simulink model "Three_Phase_180"  (R2019b)
settings: Solver=VariableStepAuto  StartTime=0.0  StopTime=0.1  RelTol=1e-3
libraries: powerlib x17
settings Model: Creator=swaga  LastModifiedBy=swaga
settings DataIOCC: ReturnWorkspaceOutputs=off

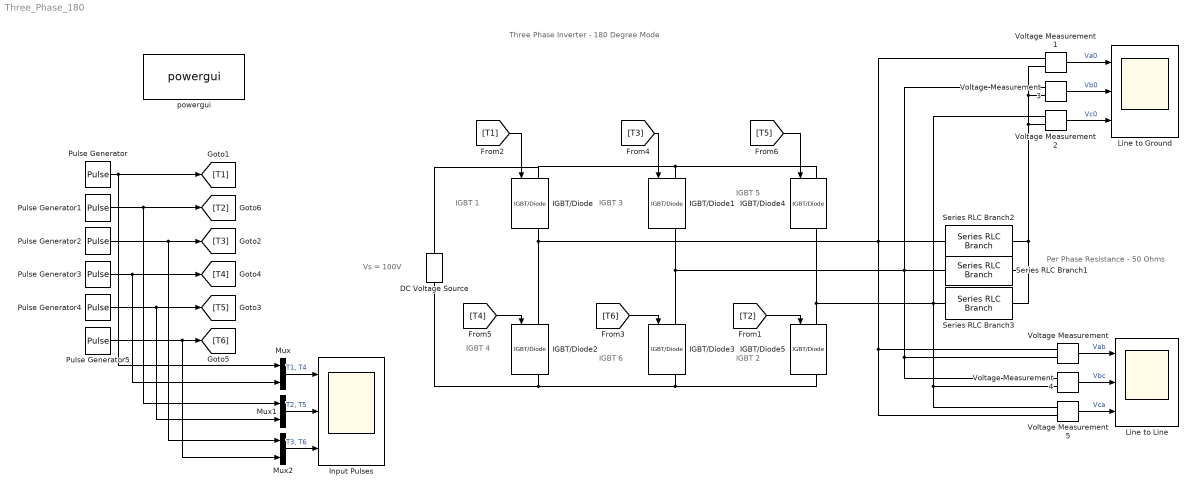
== system Three_Phase_180 ==
  note: Per Phase Resistance - 50 Ohms
  note: Vs = 100V
  note: IGBT 1
  note: Three Phase Inverter - 180 Degree Mode
  note: IGBT 3
  note: IGBT 4
  note: IGBT 6
  note: IGBT 5
  note: IGBT 2
  DC Voltage Source : powerlib/Electrical Sources/DC Voltage Source  Amplitude=100  Measurements=None
      settings: SourceProductName=Simscape Electrical
  IGBT/Diode{,1..5} (6 alike) : powerlib/Power Electronics/IGBT//Diode  Ron=1e-3  Rs=1e5  Cs=inf  Measurements=on
      settings: SourceProductName=Simscape Electrical
  Input Pulses : Scope  NumInputPorts=3
  "Line to Ground " : Scope  NumInputPorts=3
  Line to Line : Scope  NumInputPorts=3
  Mux : Mux  Inputs=2
  Mux1 : Mux  Inputs=2
  Mux2 : Mux  Inputs=2
  Pulse Generator : DiscretePulseGenerator  PulseType=Time based  Period=0.02  PulseWidth=(180/360)*100  PhaseDelay=(0/360)*0.02
  Pulse Generator1 : DiscretePulseGenerator  PulseType=Time based  Period=0.02  PulseWidth=(180/360)*100  PhaseDelay=(60/360)*0.02
  Pulse Generator2 : DiscretePulseGenerator  PulseType=Time based  Period=0.02  PulseWidth=(180/360)*100  PhaseDelay=(120/360)*0.02
  Pulse Generator3 : DiscretePulseGenerator  PulseType=Time based  Period=0.02  PulseWidth=(180/360)*100  PhaseDelay=(180/360)*0.02
  Pulse Generator4 : DiscretePulseGenerator  PulseType=Time based  Period=0.02  PulseWidth=(180/360)*100  PhaseDelay=(240/360)*0.02
  Pulse Generator5 : DiscretePulseGenerator  PulseType=Time based  Period=0.02  PulseWidth=(180/360)*100  PhaseDelay=(300/360)*0.02
  Series RLC Branch1 : powerlib/Elements/Series RLC Branch  LConnTagsString=__new0  RConnTagsString=__new0  BranchType=R  Resistance=50  Inductance=150e-6  SetiL0=off  InitialCurrent=0  Capacitance=1e-6  Setx0=off  InitialVoltage=0  Measurements=None
      settings: SourceProductName=Simscape Electrical
  Series RLC Branch2 : powerlib/Elements/Series RLC Branch  LConnTagsString=__new0  RConnTagsString=__new0  BranchType=R  Resistance=50  Inductance=150e-6  SetiL0=off  InitialCurrent=0  Capacitance=1e-6  Setx0=off  InitialVoltage=0  Measurements=None
      settings: SourceProductName=Simscape Electrical
  Series RLC Branch3 : powerlib/Elements/Series RLC Branch  LConnTagsString=__new0  RConnTagsString=__new0  BranchType=R  Resistance=50  Inductance=150e-6  SetiL0=off  InitialCurrent=0  Capacitance=1e-6  Setx0=off  InitialVoltage=0  Measurements=None
      settings: SourceProductName=Simscape Electrical
  Voltage Measurement{,1..5} (6 alike) : powerlib/Measurements/Voltage Measurement  PhasorSimulation=off  OutputType=Complex  PSBequivalent=0
      settings: SourceProductName=Simscape Electrical
  powergui : powerlib/powergui  Priority=1  SimulationMode=Continuous  SampleTime=50e-6  frequency=60  Iterations=50  frequencyindice=0  Pbase=100e6  ErrMax=1e-4  UnitsV=kV  UnitsW=MW  buscounter=0  FunctionMessages=off  echomessages=off  EnableUseOfTLC=off  CurrentSourceSwitches=off  DisableSnubberDevices=off  DisableRonSwitches=off  DisableVfSwitches=off  DisplayEquations=off  AutomaticDiscreteSolvers=off  SolverType=Tustin/Backward Euler (TBE)  Interpol=off  ExternalGateDelay=off  methode=off  Ts=100  x0status=blocks  SPID=on  SwTol=0  HookPort=off  NonlinearTolerance=1e-4  nMaxIteration=100  ContinueOnMaxIteration=off  RestoreLinks=warning  ResistiveCurrentMeasurement=off  Frange=[0:2:500]  Ylog=off  Xlog=on  ShowGrid=off  save=off  variable=ZData  structure=ScopeData  ZoomFFT=off  StartTime=0.0  cycles=1  DisplayStyle=1  fundamental=60  FreqAxis=off  MaxFrequency=1000  frequencyindicesteady=1  RmsSteady=1  display=off
      settings: SourceProductName=Simscape Electrical
  wires:
  [T4] -> IGBT/Diode2/1
  [T6] -> IGBT/Diode3/1
  [T1] -> IGBT/Diode/1
  [T3] -> IGBT/Diode1/1
  [T2] -> IGBT/Diode5/1
  [T5] -> IGBT/Diode4/1
  Pulse Generator/1 -> Mux/1, [T1]
  Pulse Generator2/1 -> Mux2/1, [T3]
  Pulse Generator3/1 -> Mux/2, [T4]
  Pulse Generator5/1 -> Mux2/2, [T6]
  Pulse Generator1/1 -> Mux1/1, [T2]
  Pulse Generator4/1 -> Mux1/2, [T5]
  Voltage Measurement4/1 -> Line to Line/2  "Vbc"
  Voltage Measurement5/1 -> Line to Line/3  "Vca"
  Voltage Measurement2/1 -> "Line to Ground "/3  "Vc0"
  Voltage Measurement3/1 -> "Line to Ground "/2  "Vb0"
  Voltage Measurement/1 -> Line to Line/1  "Vab"
  Voltage Measurement1/1 -> "Line to Ground "/1  "Va0"
  Mux1/1 -> Input Pulses/2  "T2, T5"
  Mux2/1 -> Input Pulses/3  "T3, T6"
  Mux/1 -> Input Pulses/1  "T1, T4"
  connections:
  IGBT/Diode/RConn1 -- IGBT/Diode2/LConn1 -- Voltage Measurement1/LConn1 -- Series RLC Branch2/LConn1 -- Voltage Measurement5/LConn2 -- Voltage Measurement/LConn1
  DC Voltage Source/RConn1 -- IGBT/Diode/LConn1 -- IGBT/Diode4/LConn1 -- IGBT/Diode1/LConn1
  IGBT/Diode1/RConn1 -- Series RLC Branch1/LConn1 -- Voltage Measurement4/LConn1 -- Voltage Measurement/LConn2 -- Voltage Measurement3/LConn1 -- IGBT/Diode3/LConn1
  DC Voltage Source/LConn1 -- IGBT/Diode2/RConn1 -- IGBT/Diode5/RConn1 -- IGBT/Diode3/RConn1
  IGBT/Diode4/RConn1 -- IGBT/Diode5/LConn1 -- Series RLC Branch3/LConn1 -- Voltage Measurement5/LConn1 -- Voltage Measurement4/LConn2 -- Voltage Measurement2/LConn1
  Series RLC Branch1/RConn1 -- Series RLC Branch3/RConn1 -- Series RLC Branch2/RConn1 -- Voltage Measurement3/LConn2 -- Voltage Measurement1/LConn2 -- Voltage Measurement2/LConn2
